simulink model "canLiveReaderModel"  (R2018a)
settings: Solver=FixedStepDiscrete  StartTime=0.0  StopTime=50000  RelTol=1e-3  EnableMultiTasking=on
undefined symbols (not defined in the file or in its folder): canChannel
libraries: simulink x30, canmsglib x15, canlib x5
(part 2 of 2)

== system canLiveReaderModel/CAN Information Output/Targets 0-9/Subsystem/Information Target 8/Check Target Format ==
  CAN Message : Inport
  Compare To Constant1 : simulink/Logic and Bit Operations/Compare To Constant  relop===  const=2  OutDataTypeStr=boolean
  Compare To Constant2 : simulink/Logic and Bit Operations/Compare To Constant  relop===  const=1  OutDataTypeStr=boolean
  Compare To Constant3 : simulink/Logic and Bit Operations/Compare To Constant  relop===  const=3  OutDataTypeStr=boolean
  Divide by 16 : Subsystem
  Selector4 : Selector  IndexMode=Zero-based  InputPortWidth=8  IndexOptions=Index vector (dialog)  Indices=6  OutputSizes=1
  Is format 1? : Outport
  Is format 2? : Outport  Port=2
  Is format 3? : Outport  Port=3
  wires:
  Divide by 16/1(Result) -> Compare To Constant3/1, Compare To Constant2/1, Compare To Constant1/1
  CAN Message/1 -> Selector4/1
  Selector4/1 -> Divide by 16/1(Dividend)
  Compare To Constant1/1 -> Is format 2?/1
  Compare To Constant2/1 -> Is format 1?/1
  Compare To Constant3/1 -> Is format 3?/1

== system canLiveReaderModel/CAN Information Output/Targets 0-9/Subsystem/Information Target 8/Target Format 2 ==
  CAN Message : Inport
  Enable : EnablePort
  Bearing : Subsystem
  Range : Subsystem
  Range (m) : Outport
  Bearing (°) : Outport  Port=2
  wires:
  CAN Message/1 -> Bearing/1(CAN Message), Range/1(CAN Message)
  Range/1(Range (m)) -> Range (m)/1
  Bearing/1(Bearing (°)) -> Bearing (°)/1

== system canLiveReaderModel/CAN Information Output/Targets 0-9/Subsystem/Information Target 9/Check Target Format ==
  CAN Message : Inport
  Compare To Constant1 : simulink/Logic and Bit Operations/Compare To Constant  relop===  const=2  OutDataTypeStr=boolean
  Compare To Constant2 : simulink/Logic and Bit Operations/Compare To Constant  relop===  const=1  OutDataTypeStr=boolean
  Compare To Constant3 : simulink/Logic and Bit Operations/Compare To Constant  relop===  const=3  OutDataTypeStr=boolean
  Divide by 16 : Subsystem
  Selector4 : Selector  IndexMode=Zero-based  InputPortWidth=8  IndexOptions=Index vector (dialog)  Indices=6  OutputSizes=1
  Is format 1? : Outport
  Is format 2? : Outport  Port=2
  Is format 3? : Outport  Port=3
  wires:
  Divide by 16/1(Result) -> Compare To Constant3/1, Compare To Constant2/1, Compare To Constant1/1
  CAN Message/1 -> Selector4/1
  Selector4/1 -> Divide by 16/1(Dividend)
  Compare To Constant1/1 -> Is format 2?/1
  Compare To Constant2/1 -> Is format 1?/1
  Compare To Constant3/1 -> Is format 3?/1

== system canLiveReaderModel/CAN Information Output/Targets 0-9/Subsystem/Information Target 9/Target Format 2 ==
  CAN Message : Inport
  Enable : EnablePort
  Bearing : Subsystem
  Range : Subsystem
  Range (m) : Outport
  Bearing (°) : Outport  Port=2
  wires:
  CAN Message/1 -> Bearing/1(CAN Message), Range/1(CAN Message)
  Range/1(Range (m)) -> Range (m)/1
  Bearing/1(Bearing (°)) -> Bearing (°)/1

== system canLiveReaderModel/CAN Information Output/Targets 0-9/Subsystem/Information Target 0/Check Target Format/Divide by 16 ==
  Dividend : Inport
  Constant1 : Constant  Value=16  OutDataTypeStr=Inherit: Inherit via back propagation
  Divide : Product  Inputs=*/
  Result : Outport
  wires:
  Constant1/1 -> Divide/2
  Dividend/1 -> Divide/1
  Divide/1 -> Result/1

== system canLiveReaderModel/CAN Information Output/Targets 0-9/Subsystem/Information Target 0/Target Format 2/Bearing ==
  CAN Message : Inport
  Divide by 5 : Subsystem
  Gain1 : Gain  Gain=256  OutDataTypeStr=uint16
  Gain2 : Gain  OutDataTypeStr=uint16
  Mod 4 : Subsystem
  Selector2 : Selector  IndexMode=Zero-based  InputPortWidth=8  IndexOptions=Index vector (dialog)  Indices=2  OutputSizes=1
  Selector3 : Selector  IndexMode=Zero-based  InputPortWidth=8  IndexOptions=Index vector (dialog)  Indices=3  OutputSizes=1
  Sum1 : Sum  Inputs=|++|  OutMin=-512  OutMax=511  OutDataTypeStr=fixdt(1,10,0)  InputSameDT=on
  Bearing (°) : Outport
  wires:
  Sum1/1 -> Divide by 5/1(Dividend)
  Gain2/1 -> Sum1/2
  Mod 4/1(Output) -> Gain1/1
  Gain1/1 -> Sum1/1
  CAN Message/1 -> Selector3/1, Selector2/1
  Divide by 5/1(Result) -> Bearing (°)/1
  Selector3/1 -> Gain2/1
  Selector2/1 -> Mod 4/1(Input)

== system canLiveReaderModel/CAN Information Output/Targets 0-9/Subsystem/Information Target 0/Target Format 2/Range ==
  CAN Message : Inport
  Divide by 100 : Subsystem
  Divide by 16 : Subsystem
  Gain : Gain  Gain=16  OutDataTypeStr=uint16
  Selector : Selector  IndexMode=Zero-based  InputPortWidth=8  IndexOptions=Index vector (dialog)  Indices=1  OutputSizes=1
  Selector1 : Selector  IndexMode=Zero-based  InputPortWidth=8  IndexOptions=Index vector (dialog)  Indices=0  OutputSizes=1
  Sum : Sum  Inputs=|++|  AccumDataTypeStr=uint16  InputSameDT=on
  Range (m) : Outport
  wires:
  Selector/1 -> Divide by 16/1(Dividend)
  Sum/1 -> Divide by 100/1(Dividend)
  Divide by 16/1(Result) -> Sum/2
  Divide by 100/1(Result) -> Range (m)/1
  CAN Message/1 -> Selector/1, Selector1/1
  Selector1/1 -> Gain/1
  Gain/1 -> Sum/1

== system canLiveReaderModel/CAN Information Output/Targets 0-9/Subsystem/Information Target 1/Check Target Format/Divide by 16 ==
  Dividend : Inport
  Constant1 : Constant  Value=16  OutDataTypeStr=Inherit: Inherit via back propagation
  Divide : Product  Inputs=*/
  Result : Outport
  wires:
  Constant1/1 -> Divide/2
  Dividend/1 -> Divide/1
  Divide/1 -> Result/1

== system canLiveReaderModel/CAN Information Output/Targets 0-9/Subsystem/Information Target 1/Target Format 2/Bearing ==
  CAN Message : Inport
  Divide by 5 : Subsystem
  Gain1 : Gain  Gain=256  OutDataTypeStr=uint16
  Gain2 : Gain  OutDataTypeStr=uint16
  Mod 4 : Subsystem
  Selector2 : Selector  IndexMode=Zero-based  InputPortWidth=8  IndexOptions=Index vector (dialog)  Indices=2  OutputSizes=1
  Selector3 : Selector  IndexMode=Zero-based  InputPortWidth=8  IndexOptions=Index vector (dialog)  Indices=3  OutputSizes=1
  Sum1 : Sum  Inputs=|++|  OutMin=-512  OutMax=511  OutDataTypeStr=fixdt(1,10,0)  InputSameDT=on
  Bearing (°) : Outport
  wires:
  Sum1/1 -> Divide by 5/1(Dividend)
  Gain2/1 -> Sum1/2
  Mod 4/1(Output) -> Gain1/1
  Gain1/1 -> Sum1/1
  CAN Message/1 -> Selector3/1, Selector2/1
  Divide by 5/1(Result) -> Bearing (°)/1
  Selector3/1 -> Gain2/1
  Selector2/1 -> Mod 4/1(Input)

== system canLiveReaderModel/CAN Information Output/Targets 0-9/Subsystem/Information Target 1/Target Format 2/Range ==
  CAN Message : Inport
  Divide by 100 : Subsystem
  Divide by 16 : Subsystem
  Gain : Gain  Gain=16  OutDataTypeStr=uint16
  Selector : Selector  IndexMode=Zero-based  InputPortWidth=8  IndexOptions=Index vector (dialog)  Indices=1  OutputSizes=1
  Selector1 : Selector  IndexMode=Zero-based  InputPortWidth=8  IndexOptions=Index vector (dialog)  Indices=0  OutputSizes=1
  Sum : Sum  Inputs=|++|  AccumDataTypeStr=uint16  InputSameDT=on
  Range (m) : Outport
  wires:
  Selector/1 -> Divide by 16/1(Dividend)
  Sum/1 -> Divide by 100/1(Dividend)
  Divide by 16/1(Result) -> Sum/2
  Divide by 100/1(Result) -> Range (m)/1
  CAN Message/1 -> Selector/1, Selector1/1
  Selector1/1 -> Gain/1
  Gain/1 -> Sum/1

== system canLiveReaderModel/CAN Information Output/Targets 0-9/Subsystem/Information Target 2/Check Target Format/Divide by 16 ==
  Dividend : Inport
  Constant1 : Constant  Value=16  OutDataTypeStr=Inherit: Inherit via back propagation
  Divide : Product  Inputs=*/
  Result : Outport
  wires:
  Constant1/1 -> Divide/2
  Dividend/1 -> Divide/1
  Divide/1 -> Result/1

== system canLiveReaderModel/CAN Information Output/Targets 0-9/Subsystem/Information Target 2/Target Format 2/Bearing ==
  CAN Message : Inport
  Divide by 5 : Subsystem
  Gain1 : Gain  Gain=256  OutDataTypeStr=uint16
  Gain2 : Gain  OutDataTypeStr=uint16
  Mod 4 : Subsystem
  Selector2 : Selector  IndexMode=Zero-based  InputPortWidth=8  IndexOptions=Index vector (dialog)  Indices=2  OutputSizes=1
  Selector3 : Selector  IndexMode=Zero-based  InputPortWidth=8  IndexOptions=Index vector (dialog)  Indices=3  OutputSizes=1
  Sum1 : Sum  Inputs=|++|  OutMin=-512  OutMax=511  OutDataTypeStr=fixdt(1,10,0)  InputSameDT=on
  Bearing (°) : Outport
  wires:
  Sum1/1 -> Divide by 5/1(Dividend)
  Gain2/1 -> Sum1/2
  Mod 4/1(Output) -> Gain1/1
  Gain1/1 -> Sum1/1
  CAN Message/1 -> Selector3/1, Selector2/1
  Divide by 5/1(Result) -> Bearing (°)/1
  Selector3/1 -> Gain2/1
  Selector2/1 -> Mod 4/1(Input)

== system canLiveReaderModel/CAN Information Output/Targets 0-9/Subsystem/Information Target 2/Target Format 2/Range ==
  CAN Message : Inport
  Divide by 100 : Subsystem
  Divide by 16 : Subsystem
  Gain : Gain  Gain=16  OutDataTypeStr=uint16
  Selector : Selector  IndexMode=Zero-based  InputPortWidth=8  IndexOptions=Index vector (dialog)  Indices=1  OutputSizes=1
  Selector1 : Selector  IndexMode=Zero-based  InputPortWidth=8  IndexOptions=Index vector (dialog)  Indices=0  OutputSizes=1
  Sum : Sum  Inputs=|++|  AccumDataTypeStr=uint16  InputSameDT=on
  Range (m) : Outport
  wires:
  Selector/1 -> Divide by 16/1(Dividend)
  Sum/1 -> Divide by 100/1(Dividend)
  Divide by 16/1(Result) -> Sum/2
  Divide by 100/1(Result) -> Range (m)/1
  CAN Message/1 -> Selector/1, Selector1/1
  Selector1/1 -> Gain/1
  Gain/1 -> Sum/1

== system canLiveReaderModel/CAN Information Output/Targets 0-9/Subsystem/Information Target 3/Check Target Format/Divide by 16 ==
  Dividend : Inport
  Constant1 : Constant  Value=16  OutDataTypeStr=Inherit: Inherit via back propagation
  Divide : Product  Inputs=*/
  Result : Outport
  wires:
  Constant1/1 -> Divide/2
  Dividend/1 -> Divide/1
  Divide/1 -> Result/1

== system canLiveReaderModel/CAN Information Output/Targets 0-9/Subsystem/Information Target 3/Target Format 2/Bearing ==
  CAN Message : Inport
  Divide by 5 : Subsystem
  Gain1 : Gain  Gain=256  OutDataTypeStr=uint16
  Gain2 : Gain  OutDataTypeStr=uint16
  Mod 4 : Subsystem
  Selector2 : Selector  IndexMode=Zero-based  InputPortWidth=8  IndexOptions=Index vector (dialog)  Indices=2  OutputSizes=1
  Selector3 : Selector  IndexMode=Zero-based  InputPortWidth=8  IndexOptions=Index vector (dialog)  Indices=3  OutputSizes=1
  Sum1 : Sum  Inputs=|++|  OutMin=-512  OutMax=511  OutDataTypeStr=fixdt(1,10,0)  InputSameDT=on
  Bearing (°) : Outport
  wires:
  Sum1/1 -> Divide by 5/1(Dividend)
  Gain2/1 -> Sum1/2
  Mod 4/1(Output) -> Gain1/1
  Gain1/1 -> Sum1/1
  CAN Message/1 -> Selector3/1, Selector2/1
  Divide by 5/1(Result) -> Bearing (°)/1
  Selector3/1 -> Gain2/1
  Selector2/1 -> Mod 4/1(Input)

== system canLiveReaderModel/CAN Information Output/Targets 0-9/Subsystem/Information Target 3/Target Format 2/Range ==
  CAN Message : Inport
  Divide by 100 : Subsystem
  Divide by 16 : Subsystem
  Gain : Gain  Gain=16  OutDataTypeStr=uint16
  Selector : Selector  IndexMode=Zero-based  InputPortWidth=8  IndexOptions=Index vector (dialog)  Indices=1  OutputSizes=1
  Selector1 : Selector  IndexMode=Zero-based  InputPortWidth=8  IndexOptions=Index vector (dialog)  Indices=0  OutputSizes=1
  Sum : Sum  Inputs=|++|  AccumDataTypeStr=uint16  InputSameDT=on
  Range (m) : Outport
  wires:
  Selector/1 -> Divide by 16/1(Dividend)
  Sum/1 -> Divide by 100/1(Dividend)
  Divide by 16/1(Result) -> Sum/2
  Divide by 100/1(Result) -> Range (m)/1
  CAN Message/1 -> Selector/1, Selector1/1
  Selector1/1 -> Gain/1
  Gain/1 -> Sum/1

== system canLiveReaderModel/CAN Information Output/Targets 0-9/Subsystem/Information Target 4/Check Target Format/Divide by 16 ==
  Dividend : Inport
  Constant1 : Constant  Value=16  OutDataTypeStr=Inherit: Inherit via back propagation
  Divide : Product  Inputs=*/
  Result : Outport
  wires:
  Constant1/1 -> Divide/2
  Dividend/1 -> Divide/1
  Divide/1 -> Result/1

== system canLiveReaderModel/CAN Information Output/Targets 0-9/Subsystem/Information Target 4/Target Format 2/Bearing ==
  CAN Message : Inport
  Divide by 5 : Subsystem
  Gain1 : Gain  Gain=256  OutDataTypeStr=uint16
  Gain2 : Gain  OutDataTypeStr=uint16
  Mod 4 : Subsystem
  Selector2 : Selector  IndexMode=Zero-based  InputPortWidth=8  IndexOptions=Index vector (dialog)  Indices=2  OutputSizes=1
  Selector3 : Selector  IndexMode=Zero-based  InputPortWidth=8  IndexOptions=Index vector (dialog)  Indices=3  OutputSizes=1
  Sum1 : Sum  Inputs=|++|  OutMin=-512  OutMax=511  OutDataTypeStr=fixdt(1,10,0)  InputSameDT=on
  Bearing (°) : Outport
  wires:
  Sum1/1 -> Divide by 5/1(Dividend)
  Gain2/1 -> Sum1/2
  Mod 4/1(Output) -> Gain1/1
  Gain1/1 -> Sum1/1
  CAN Message/1 -> Selector3/1, Selector2/1
  Divide by 5/1(Result) -> Bearing (°)/1
  Selector3/1 -> Gain2/1
  Selector2/1 -> Mod 4/1(Input)

== system canLiveReaderModel/CAN Information Output/Targets 0-9/Subsystem/Information Target 4/Target Format 2/Range ==
  CAN Message : Inport
  Divide by 100 : Subsystem
  Divide by 16 : Subsystem
  Gain : Gain  Gain=16  OutDataTypeStr=uint16
  Selector : Selector  IndexMode=Zero-based  InputPortWidth=8  IndexOptions=Index vector (dialog)  Indices=1  OutputSizes=1
  Selector1 : Selector  IndexMode=Zero-based  InputPortWidth=8  IndexOptions=Index vector (dialog)  Indices=0  OutputSizes=1
  Sum : Sum  Inputs=|++|  AccumDataTypeStr=uint16  InputSameDT=on
  Range (m) : Outport
  wires:
  Selector/1 -> Divide by 16/1(Dividend)
  Sum/1 -> Divide by 100/1(Dividend)
  Divide by 16/1(Result) -> Sum/2
  Divide by 100/1(Result) -> Range (m)/1
  CAN Message/1 -> Selector/1, Selector1/1
  Selector1/1 -> Gain/1
  Gain/1 -> Sum/1

== system canLiveReaderModel/CAN Information Output/Targets 0-9/Subsystem/Information Target 5/Check Target Format/Divide by 16 ==
  Dividend : Inport
  Constant1 : Constant  Value=16  OutDataTypeStr=Inherit: Inherit via back propagation
  Divide : Product  Inputs=*/
  Result : Outport
  wires:
  Constant1/1 -> Divide/2
  Dividend/1 -> Divide/1
  Divide/1 -> Result/1

== system canLiveReaderModel/CAN Information Output/Targets 0-9/Subsystem/Information Target 5/Target Format 2/Bearing ==
  CAN Message : Inport
  Divide by 5 : Subsystem
  Gain1 : Gain  Gain=256  OutDataTypeStr=uint16
  Gain2 : Gain  OutDataTypeStr=uint16
  Mod 4 : Subsystem
  Selector2 : Selector  IndexMode=Zero-based  InputPortWidth=8  IndexOptions=Index vector (dialog)  Indices=2  OutputSizes=1
  Selector3 : Selector  IndexMode=Zero-based  InputPortWidth=8  IndexOptions=Index vector (dialog)  Indices=3  OutputSizes=1
  Sum1 : Sum  Inputs=|++|  OutMin=-512  OutMax=511  OutDataTypeStr=fixdt(1,10,0)  InputSameDT=on
  Bearing (°) : Outport
  wires:
  Sum1/1 -> Divide by 5/1(Dividend)
  Gain2/1 -> Sum1/2
  Mod 4/1(Output) -> Gain1/1
  Gain1/1 -> Sum1/1
  CAN Message/1 -> Selector3/1, Selector2/1
  Divide by 5/1(Result) -> Bearing (°)/1
  Selector3/1 -> Gain2/1
  Selector2/1 -> Mod 4/1(Input)

== system canLiveReaderModel/CAN Information Output/Targets 0-9/Subsystem/Information Target 5/Target Format 2/Range ==
  CAN Message : Inport
  Divide by 100 : Subsystem
  Divide by 16 : Subsystem
  Gain : Gain  Gain=16  OutDataTypeStr=uint16
  Selector : Selector  IndexMode=Zero-based  InputPortWidth=8  IndexOptions=Index vector (dialog)  Indices=1  OutputSizes=1
  Selector1 : Selector  IndexMode=Zero-based  InputPortWidth=8  IndexOptions=Index vector (dialog)  Indices=0  OutputSizes=1
  Sum : Sum  Inputs=|++|  AccumDataTypeStr=uint16  InputSameDT=on
  Range (m) : Outport
  wires:
  Selector/1 -> Divide by 16/1(Dividend)
  Sum/1 -> Divide by 100/1(Dividend)
  Divide by 16/1(Result) -> Sum/2
  Divide by 100/1(Result) -> Range (m)/1
  CAN Message/1 -> Selector/1, Selector1/1
  Selector1/1 -> Gain/1
  Gain/1 -> Sum/1

== system canLiveReaderModel/CAN Information Output/Targets 0-9/Subsystem/Information Target 6/Check Target Format/Divide by 16 ==
  Dividend : Inport
  Constant1 : Constant  Value=16  OutDataTypeStr=Inherit: Inherit via back propagation
  Divide : Product  Inputs=*/
  Result : Outport
  wires:
  Constant1/1 -> Divide/2
  Dividend/1 -> Divide/1
  Divide/1 -> Result/1

== system canLiveReaderModel/CAN Information Output/Targets 0-9/Subsystem/Information Target 6/Target Format 2/Bearing ==
  CAN Message : Inport
  Divide by 5 : Subsystem
  Gain1 : Gain  Gain=256  OutDataTypeStr=uint16
  Gain2 : Gain  OutDataTypeStr=uint16
  Mod 4 : Subsystem
  Selector2 : Selector  IndexMode=Zero-based  InputPortWidth=8  IndexOptions=Index vector (dialog)  Indices=2  OutputSizes=1
  Selector3 : Selector  IndexMode=Zero-based  InputPortWidth=8  IndexOptions=Index vector (dialog)  Indices=3  OutputSizes=1
  Sum1 : Sum  Inputs=|++|  OutMin=-512  OutMax=511  OutDataTypeStr=fixdt(1,10,0)  InputSameDT=on
  Bearing (°) : Outport
  wires:
  Sum1/1 -> Divide by 5/1(Dividend)
  Gain2/1 -> Sum1/2
  Mod 4/1(Output) -> Gain1/1
  Gain1/1 -> Sum1/1
  CAN Message/1 -> Selector3/1, Selector2/1
  Divide by 5/1(Result) -> Bearing (°)/1
  Selector3/1 -> Gain2/1
  Selector2/1 -> Mod 4/1(Input)

== system canLiveReaderModel/CAN Information Output/Targets 0-9/Subsystem/Information Target 6/Target Format 2/Range ==
  CAN Message : Inport
  Divide by 100 : Subsystem
  Divide by 16 : Subsystem
  Gain : Gain  Gain=16  OutDataTypeStr=uint16
  Selector : Selector  IndexMode=Zero-based  InputPortWidth=8  IndexOptions=Index vector (dialog)  Indices=1  OutputSizes=1
  Selector1 : Selector  IndexMode=Zero-based  InputPortWidth=8  IndexOptions=Index vector (dialog)  Indices=0  OutputSizes=1
  Sum : Sum  Inputs=|++|  AccumDataTypeStr=uint16  InputSameDT=on
  Range (m) : Outport
  wires:
  Selector/1 -> Divide by 16/1(Dividend)
  Sum/1 -> Divide by 100/1(Dividend)
  Divide by 16/1(Result) -> Sum/2
  Divide by 100/1(Result) -> Range (m)/1
  CAN Message/1 -> Selector/1, Selector1/1
  Selector1/1 -> Gain/1
  Gain/1 -> Sum/1

== system canLiveReaderModel/CAN Information Output/Targets 0-9/Subsystem/Information Target 7/Check Target Format/Divide by 16 ==
  Dividend : Inport
  Constant1 : Constant  Value=16  OutDataTypeStr=Inherit: Inherit via back propagation
  Divide : Product  Inputs=*/
  Result : Outport
  wires:
  Constant1/1 -> Divide/2
  Dividend/1 -> Divide/1
  Divide/1 -> Result/1

== system canLiveReaderModel/CAN Information Output/Targets 0-9/Subsystem/Information Target 7/Target Format 2/Bearing ==
  CAN Message : Inport
  Divide by 5 : Subsystem
  Gain1 : Gain  Gain=256  OutDataTypeStr=uint16
  Gain2 : Gain  OutDataTypeStr=uint16
  Mod 4 : Subsystem
  Selector2 : Selector  IndexMode=Zero-based  InputPortWidth=8  IndexOptions=Index vector (dialog)  Indices=2  OutputSizes=1
  Selector3 : Selector  IndexMode=Zero-based  InputPortWidth=8  IndexOptions=Index vector (dialog)  Indices=3  OutputSizes=1
  Sum1 : Sum  Inputs=|++|  OutMin=-512  OutMax=511  OutDataTypeStr=fixdt(1,10,0)  InputSameDT=on
  Bearing (°) : Outport
  wires:
  Sum1/1 -> Divide by 5/1(Dividend)
  Gain2/1 -> Sum1/2
  Mod 4/1(Output) -> Gain1/1
  Gain1/1 -> Sum1/1
  CAN Message/1 -> Selector3/1, Selector2/1
  Divide by 5/1(Result) -> Bearing (°)/1
  Selector3/1 -> Gain2/1
  Selector2/1 -> Mod 4/1(Input)

== system canLiveReaderModel/CAN Information Output/Targets 0-9/Subsystem/Information Target 7/Target Format 2/Range ==
  CAN Message : Inport
  Divide by 100 : Subsystem
  Divide by 16 : Subsystem
  Gain : Gain  Gain=16  OutDataTypeStr=uint16
  Selector : Selector  IndexMode=Zero-based  InputPortWidth=8  IndexOptions=Index vector (dialog)  Indices=1  OutputSizes=1
  Selector1 : Selector  IndexMode=Zero-based  InputPortWidth=8  IndexOptions=Index vector (dialog)  Indices=0  OutputSizes=1
  Sum : Sum  Inputs=|++|  AccumDataTypeStr=uint16  InputSameDT=on
  Range (m) : Outport
  wires:
  Selector/1 -> Divide by 16/1(Dividend)
  Sum/1 -> Divide by 100/1(Dividend)
  Divide by 16/1(Result) -> Sum/2
  Divide by 100/1(Result) -> Range (m)/1
  CAN Message/1 -> Selector/1, Selector1/1
  Selector1/1 -> Gain/1
  Gain/1 -> Sum/1

== system canLiveReaderModel/CAN Information Output/Targets 0-9/Subsystem/Information Target 8/Check Target Format/Divide by 16 ==
  Dividend : Inport
  Constant1 : Constant  Value=16  OutDataTypeStr=Inherit: Inherit via back propagation
  Divide : Product  Inputs=*/
  Result : Outport
  wires:
  Constant1/1 -> Divide/2
  Dividend/1 -> Divide/1
  Divide/1 -> Result/1

== system canLiveReaderModel/CAN Information Output/Targets 0-9/Subsystem/Information Target 8/Target Format 2/Bearing ==
  CAN Message : Inport
  Divide by 5 : Subsystem
  Gain1 : Gain  Gain=256  OutDataTypeStr=uint16
  Gain2 : Gain  OutDataTypeStr=uint16
  Mod 4 : Subsystem
  Selector2 : Selector  IndexMode=Zero-based  InputPortWidth=8  IndexOptions=Index vector (dialog)  Indices=2  OutputSizes=1
  Selector3 : Selector  IndexMode=Zero-based  InputPortWidth=8  IndexOptions=Index vector (dialog)  Indices=3  OutputSizes=1
  Sum1 : Sum  Inputs=|++|  OutMin=-512  OutMax=511  OutDataTypeStr=fixdt(1,10,0)  InputSameDT=on
  Bearing (°) : Outport
  wires:
  Sum1/1 -> Divide by 5/1(Dividend)
  Gain2/1 -> Sum1/2
  Mod 4/1(Output) -> Gain1/1
  Gain1/1 -> Sum1/1
  CAN Message/1 -> Selector3/1, Selector2/1
  Divide by 5/1(Result) -> Bearing (°)/1
  Selector3/1 -> Gain2/1
  Selector2/1 -> Mod 4/1(Input)

== system canLiveReaderModel/CAN Information Output/Targets 0-9/Subsystem/Information Target 8/Target Format 2/Range ==
  CAN Message : Inport
  Divide by 100 : Subsystem
  Divide by 16 : Subsystem
  Gain : Gain  Gain=16  OutDataTypeStr=uint16
  Selector : Selector  IndexMode=Zero-based  InputPortWidth=8  IndexOptions=Index vector (dialog)  Indices=1  OutputSizes=1
  Selector1 : Selector  IndexMode=Zero-based  InputPortWidth=8  IndexOptions=Index vector (dialog)  Indices=0  OutputSizes=1
  Sum : Sum  Inputs=|++|  AccumDataTypeStr=uint16  InputSameDT=on
  Range (m) : Outport
  wires:
  Selector/1 -> Divide by 16/1(Dividend)
  Sum/1 -> Divide by 100/1(Dividend)
  Divide by 16/1(Result) -> Sum/2
  Divide by 100/1(Result) -> Range (m)/1
  CAN Message/1 -> Selector/1, Selector1/1
  Selector1/1 -> Gain/1
  Gain/1 -> Sum/1

== system canLiveReaderModel/CAN Information Output/Targets 0-9/Subsystem/Information Target 9/Check Target Format/Divide by 16 ==
  Dividend : Inport
  Constant1 : Constant  Value=16  OutDataTypeStr=Inherit: Inherit via back propagation
  Divide : Product  Inputs=*/
  Result : Outport
  wires:
  Constant1/1 -> Divide/2
  Dividend/1 -> Divide/1
  Divide/1 -> Result/1

== system canLiveReaderModel/CAN Information Output/Targets 0-9/Subsystem/Information Target 9/Target Format 2/Bearing ==
  CAN Message : Inport
  Divide by 5 : Subsystem
  Gain1 : Gain  Gain=256  OutDataTypeStr=uint16
  Gain2 : Gain  OutDataTypeStr=uint16
  Mod 4 : Subsystem
  Selector2 : Selector  IndexMode=Zero-based  InputPortWidth=8  IndexOptions=Index vector (dialog)  Indices=2  OutputSizes=1
  Selector3 : Selector  IndexMode=Zero-based  InputPortWidth=8  IndexOptions=Index vector (dialog)  Indices=3  OutputSizes=1
  Sum1 : Sum  Inputs=|++|  OutMin=-512  OutMax=511  OutDataTypeStr=fixdt(1,10,0)  InputSameDT=on
  Bearing (°) : Outport
  wires:
  Sum1/1 -> Divide by 5/1(Dividend)
  Gain2/1 -> Sum1/2
  Mod 4/1(Output) -> Gain1/1
  Gain1/1 -> Sum1/1
  CAN Message/1 -> Selector3/1, Selector2/1
  Divide by 5/1(Result) -> Bearing (°)/1
  Selector3/1 -> Gain2/1
  Selector2/1 -> Mod 4/1(Input)

== system canLiveReaderModel/CAN Information Output/Targets 0-9/Subsystem/Information Target 9/Target Format 2/Range ==
  CAN Message : Inport
  Divide by 100 : Subsystem
  Divide by 16 : Subsystem
  Gain : Gain  Gain=16  OutDataTypeStr=uint16
  Selector : Selector  IndexMode=Zero-based  InputPortWidth=8  IndexOptions=Index vector (dialog)  Indices=1  OutputSizes=1
  Selector1 : Selector  IndexMode=Zero-based  InputPortWidth=8  IndexOptions=Index vector (dialog)  Indices=0  OutputSizes=1
  Sum : Sum  Inputs=|++|  AccumDataTypeStr=uint16  InputSameDT=on
  Range (m) : Outport
  wires:
  Selector/1 -> Divide by 16/1(Dividend)
  Sum/1 -> Divide by 100/1(Dividend)
  Divide by 16/1(Result) -> Sum/2
  Divide by 100/1(Result) -> Range (m)/1
  CAN Message/1 -> Selector/1, Selector1/1
  Selector1/1 -> Gain/1
  Gain/1 -> Sum/1

== system canLiveReaderModel/CAN Information Output/Targets 0-9/Subsystem/Information Target 0/Target Format 2/Bearing/Divide by 5 ==
  Dividend : Inport
  Constant1 : Constant  Value=5  OutDataTypeStr=Inherit: Inherit via back propagation
  Divide : Product  Inputs=*/  OutDataTypeStr=double
  Result : Outport
  wires:
  Constant1/1 -> Divide/2
  Divide/1 -> Result/1
  Dividend/1 -> Divide/1

== system canLiveReaderModel/CAN Information Output/Targets 0-9/Subsystem/Information Target 0/Target Format 2/Bearing/Mod 4 ==
  Input : Inport
  Constant : Constant  Value=4  OutDataTypeStr=Inherit: Inherit via back propagation
  Rem : Math  Operator=mod  OutputSignalType=real  SaturateOnIntegerOverflow=on
  Output : Outport
  wires:
  Input/1 -> Rem/1
  Constant/1 -> Rem/2
  Rem/1 -> Output/1

== system canLiveReaderModel/CAN Information Output/Targets 0-9/Subsystem/Information Target 0/Target Format 2/Range/Divide by 100 ==
  Dividend : Inport
  Constant1 : Constant  Value=100  OutDataTypeStr=Inherit: Inherit via back propagation
  Divide : Product  Inputs=*/  OutDataTypeStr=double
  Result : Outport
  wires:
  Constant1/1 -> Divide/2
  Divide/1 -> Result/1
  Dividend/1 -> Divide/1

== system canLiveReaderModel/CAN Information Output/Targets 0-9/Subsystem/Information Target 0/Target Format 2/Range/Divide by 16 ==
  Dividend : Inport
  Constant1 : Constant  Value=16  OutDataTypeStr=Inherit: Inherit via back propagation
  Divide : Product  Inputs=*/
  Result : Outport
  wires:
  Constant1/1 -> Divide/2
  Dividend/1 -> Divide/1
  Divide/1 -> Result/1

== system canLiveReaderModel/CAN Information Output/Targets 0-9/Subsystem/Information Target 1/Target Format 2/Bearing/Divide by 5 ==
  Dividend : Inport
  Constant1 : Constant  Value=5  OutDataTypeStr=Inherit: Inherit via back propagation
  Divide : Product  Inputs=*/  OutDataTypeStr=double
  Result : Outport
  wires:
  Constant1/1 -> Divide/2
  Divide/1 -> Result/1
  Dividend/1 -> Divide/1

== system canLiveReaderModel/CAN Information Output/Targets 0-9/Subsystem/Information Target 1/Target Format 2/Bearing/Mod 4 ==
  Input : Inport
  Constant : Constant  Value=4  OutDataTypeStr=Inherit: Inherit via back propagation
  Rem : Math  Operator=mod  OutputSignalType=real  SaturateOnIntegerOverflow=on
  Output : Outport
  wires:
  Input/1 -> Rem/1
  Constant/1 -> Rem/2
  Rem/1 -> Output/1

== system canLiveReaderModel/CAN Information Output/Targets 0-9/Subsystem/Information Target 1/Target Format 2/Range/Divide by 100 ==
  Dividend : Inport
  Constant1 : Constant  Value=100  OutDataTypeStr=Inherit: Inherit via back propagation
  Divide : Product  Inputs=*/  OutDataTypeStr=double
  Result : Outport
  wires:
  Constant1/1 -> Divide/2
  Divide/1 -> Result/1
  Dividend/1 -> Divide/1

== system canLiveReaderModel/CAN Information Output/Targets 0-9/Subsystem/Information Target 1/Target Format 2/Range/Divide by 16 ==
  Dividend : Inport
  Constant1 : Constant  Value=16  OutDataTypeStr=Inherit: Inherit via back propagation
  Divide : Product  Inputs=*/
  Result : Outport
  wires:
  Constant1/1 -> Divide/2
  Dividend/1 -> Divide/1
  Divide/1 -> Result/1

== system canLiveReaderModel/CAN Information Output/Targets 0-9/Subsystem/Information Target 2/Target Format 2/Bearing/Divide by 5 ==
  Dividend : Inport
  Constant1 : Constant  Value=5  OutDataTypeStr=Inherit: Inherit via back propagation
  Divide : Product  Inputs=*/  OutDataTypeStr=double
  Result : Outport
  wires:
  Constant1/1 -> Divide/2
  Divide/1 -> Result/1
  Dividend/1 -> Divide/1

== system canLiveReaderModel/CAN Information Output/Targets 0-9/Subsystem/Information Target 2/Target Format 2/Bearing/Mod 4 ==
  Input : Inport
  Constant : Constant  Value=4  OutDataTypeStr=Inherit: Inherit via back propagation
  Rem : Math  Operator=mod  OutputSignalType=real  SaturateOnIntegerOverflow=on
  Output : Outport
  wires:
  Input/1 -> Rem/1
  Constant/1 -> Rem/2
  Rem/1 -> Output/1

== system canLiveReaderModel/CAN Information Output/Targets 0-9/Subsystem/Information Target 2/Target Format 2/Range/Divide by 100 ==
  Dividend : Inport
  Constant1 : Constant  Value=100  OutDataTypeStr=Inherit: Inherit via back propagation
  Divide : Product  Inputs=*/  OutDataTypeStr=double
  Result : Outport
  wires:
  Constant1/1 -> Divide/2
  Divide/1 -> Result/1
  Dividend/1 -> Divide/1

== system canLiveReaderModel/CAN Information Output/Targets 0-9/Subsystem/Information Target 2/Target Format 2/Range/Divide by 16 ==
  Dividend : Inport
  Constant1 : Constant  Value=16  OutDataTypeStr=Inherit: Inherit via back propagation
  Divide : Product  Inputs=*/
  Result : Outport
  wires:
  Constant1/1 -> Divide/2
  Dividend/1 -> Divide/1
  Divide/1 -> Result/1

== system canLiveReaderModel/CAN Information Output/Targets 0-9/Subsystem/Information Target 3/Target Format 2/Bearing/Divide by 5 ==
  Dividend : Inport
  Constant1 : Constant  Value=5  OutDataTypeStr=Inherit: Inherit via back propagation
  Divide : Product  Inputs=*/  OutDataTypeStr=double
  Result : Outport
  wires:
  Constant1/1 -> Divide/2
  Divide/1 -> Result/1
  Dividend/1 -> Divide/1

== system canLiveReaderModel/CAN Information Output/Targets 0-9/Subsystem/Information Target 3/Target Format 2/Bearing/Mod 4 ==
  Input : Inport
  Constant : Constant  Value=4  OutDataTypeStr=Inherit: Inherit via back propagation
  Rem : Math  Operator=mod  OutputSignalType=real  SaturateOnIntegerOverflow=on
  Output : Outport
  wires:
  Input/1 -> Rem/1
  Constant/1 -> Rem/2
  Rem/1 -> Output/1

== system canLiveReaderModel/CAN Information Output/Targets 0-9/Subsystem/Information Target 3/Target Format 2/Range/Divide by 100 ==
  Dividend : Inport
  Constant1 : Constant  Value=100  OutDataTypeStr=Inherit: Inherit via back propagation
  Divide : Product  Inputs=*/  OutDataTypeStr=double
  Result : Outport
  wires:
  Constant1/1 -> Divide/2
  Divide/1 -> Result/1
  Dividend/1 -> Divide/1

== system canLiveReaderModel/CAN Information Output/Targets 0-9/Subsystem/Information Target 3/Target Format 2/Range/Divide by 16 ==
  Dividend : Inport
  Constant1 : Constant  Value=16  OutDataTypeStr=Inherit: Inherit via back propagation
  Divide : Product  Inputs=*/
  Result : Outport
  wires:
  Constant1/1 -> Divide/2
  Dividend/1 -> Divide/1
  Divide/1 -> Result/1

== system canLiveReaderModel/CAN Information Output/Targets 0-9/Subsystem/Information Target 4/Target Format 2/Bearing/Divide by 5 ==
  Dividend : Inport
  Constant1 : Constant  Value=5  OutDataTypeStr=Inherit: Inherit via back propagation
  Divide : Product  Inputs=*/  OutDataTypeStr=double
  Result : Outport
  wires:
  Constant1/1 -> Divide/2
  Divide/1 -> Result/1
  Dividend/1 -> Divide/1

== system canLiveReaderModel/CAN Information Output/Targets 0-9/Subsystem/Information Target 4/Target Format 2/Bearing/Mod 4 ==
  Input : Inport
  Constant : Constant  Value=4  OutDataTypeStr=Inherit: Inherit via back propagation
  Rem : Math  Operator=mod  OutputSignalType=real  SaturateOnIntegerOverflow=on
  Output : Outport
  wires:
  Input/1 -> Rem/1
  Constant/1 -> Rem/2
  Rem/1 -> Output/1

== system canLiveReaderModel/CAN Information Output/Targets 0-9/Subsystem/Information Target 4/Target Format 2/Range/Divide by 100 ==
  Dividend : Inport
  Constant1 : Constant  Value=100  OutDataTypeStr=Inherit: Inherit via back propagation
  Divide : Product  Inputs=*/  OutDataTypeStr=double
  Result : Outport
  wires:
  Constant1/1 -> Divide/2
  Divide/1 -> Result/1
  Dividend/1 -> Divide/1

== system canLiveReaderModel/CAN Information Output/Targets 0-9/Subsystem/Information Target 4/Target Format 2/Range/Divide by 16 ==
  Dividend : Inport
  Constant1 : Constant  Value=16  OutDataTypeStr=Inherit: Inherit via back propagation
  Divide : Product  Inputs=*/
  Result : Outport
  wires:
  Constant1/1 -> Divide/2
  Dividend/1 -> Divide/1
  Divide/1 -> Result/1

== system canLiveReaderModel/CAN Information Output/Targets 0-9/Subsystem/Information Target 5/Target Format 2/Bearing/Divide by 5 ==
  Dividend : Inport
  Constant1 : Constant  Value=5  OutDataTypeStr=Inherit: Inherit via back propagation
  Divide : Product  Inputs=*/  OutDataTypeStr=double
  Result : Outport
  wires:
  Constant1/1 -> Divide/2
  Divide/1 -> Result/1
  Dividend/1 -> Divide/1

== system canLiveReaderModel/CAN Information Output/Targets 0-9/Subsystem/Information Target 5/Target Format 2/Bearing/Mod 4 ==
  Input : Inport
  Constant : Constant  Value=4  OutDataTypeStr=Inherit: Inherit via back propagation
  Rem : Math  Operator=mod  OutputSignalType=real  SaturateOnIntegerOverflow=on
  Output : Outport
  wires:
  Input/1 -> Rem/1
  Constant/1 -> Rem/2
  Rem/1 -> Output/1

== system canLiveReaderModel/CAN Information Output/Targets 0-9/Subsystem/Information Target 5/Target Format 2/Range/Divide by 100 ==
  Dividend : Inport
  Constant1 : Constant  Value=100  OutDataTypeStr=Inherit: Inherit via back propagation
  Divide : Product  Inputs=*/  OutDataTypeStr=double
  Result : Outport
  wires:
  Constant1/1 -> Divide/2
  Divide/1 -> Result/1
  Dividend/1 -> Divide/1

== system canLiveReaderModel/CAN Information Output/Targets 0-9/Subsystem/Information Target 5/Target Format 2/Range/Divide by 16 ==
  Dividend : Inport
  Constant1 : Constant  Value=16  OutDataTypeStr=Inherit: Inherit via back propagation
  Divide : Product  Inputs=*/
  Result : Outport
  wires:
  Constant1/1 -> Divide/2
  Dividend/1 -> Divide/1
  Divide/1 -> Result/1

== system canLiveReaderModel/CAN Information Output/Targets 0-9/Subsystem/Information Target 6/Target Format 2/Bearing/Divide by 5 ==
  Dividend : Inport
  Constant1 : Constant  Value=5  OutDataTypeStr=Inherit: Inherit via back propagation
  Divide : Product  Inputs=*/  OutDataTypeStr=double
  Result : Outport
  wires:
  Constant1/1 -> Divide/2
  Divide/1 -> Result/1
  Dividend/1 -> Divide/1

== system canLiveReaderModel/CAN Information Output/Targets 0-9/Subsystem/Information Target 6/Target Format 2/Bearing/Mod 4 ==
  Input : Inport
  Constant : Constant  Value=4  OutDataTypeStr=Inherit: Inherit via back propagation
  Rem : Math  Operator=mod  OutputSignalType=real  SaturateOnIntegerOverflow=on
  Output : Outport
  wires:
  Input/1 -> Rem/1
  Constant/1 -> Rem/2
  Rem/1 -> Output/1

== system canLiveReaderModel/CAN Information Output/Targets 0-9/Subsystem/Information Target 6/Target Format 2/Range/Divide by 100 ==
  Dividend : Inport
  Constant1 : Constant  Value=100  OutDataTypeStr=Inherit: Inherit via back propagation
  Divide : Product  Inputs=*/  OutDataTypeStr=double
  Result : Outport
  wires:
  Constant1/1 -> Divide/2
  Divide/1 -> Result/1
  Dividend/1 -> Divide/1

== system canLiveReaderModel/CAN Information Output/Targets 0-9/Subsystem/Information Target 6/Target Format 2/Range/Divide by 16 ==
  Dividend : Inport
  Constant1 : Constant  Value=16  OutDataTypeStr=Inherit: Inherit via back propagation
  Divide : Product  Inputs=*/
  Result : Outport
  wires:
  Constant1/1 -> Divide/2
  Dividend/1 -> Divide/1
  Divide/1 -> Result/1

== system canLiveReaderModel/CAN Information Output/Targets 0-9/Subsystem/Information Target 7/Target Format 2/Bearing/Divide by 5 ==
  Dividend : Inport
  Constant1 : Constant  Value=5  OutDataTypeStr=Inherit: Inherit via back propagation
  Divide : Product  Inputs=*/  OutDataTypeStr=double
  Result : Outport
  wires:
  Constant1/1 -> Divide/2
  Divide/1 -> Result/1
  Dividend/1 -> Divide/1

== system canLiveReaderModel/CAN Information Output/Targets 0-9/Subsystem/Information Target 7/Target Format 2/Bearing/Mod 4 ==
  Input : Inport
  Constant : Constant  Value=4  OutDataTypeStr=Inherit: Inherit via back propagation
  Rem : Math  Operator=mod  OutputSignalType=real  SaturateOnIntegerOverflow=on
  Output : Outport
  wires:
  Input/1 -> Rem/1
  Constant/1 -> Rem/2
  Rem/1 -> Output/1

== system canLiveReaderModel/CAN Information Output/Targets 0-9/Subsystem/Information Target 7/Target Format 2/Range/Divide by 100 ==
  Dividend : Inport
  Constant1 : Constant  Value=100  OutDataTypeStr=Inherit: Inherit via back propagation
  Divide : Product  Inputs=*/  OutDataTypeStr=double
  Result : Outport
  wires:
  Constant1/1 -> Divide/2
  Divide/1 -> Result/1
  Dividend/1 -> Divide/1

== system canLiveReaderModel/CAN Information Output/Targets 0-9/Subsystem/Information Target 7/Target Format 2/Range/Divide by 16 ==
  Dividend : Inport
  Constant1 : Constant  Value=16  OutDataTypeStr=Inherit: Inherit via back propagation
  Divide : Product  Inputs=*/
  Result : Outport
  wires:
  Constant1/1 -> Divide/2
  Dividend/1 -> Divide/1
  Divide/1 -> Result/1

== system canLiveReaderModel/CAN Information Output/Targets 0-9/Subsystem/Information Target 8/Target Format 2/Bearing/Divide by 5 ==
  Dividend : Inport
  Constant1 : Constant  Value=5  OutDataTypeStr=Inherit: Inherit via back propagation
  Divide : Product  Inputs=*/  OutDataTypeStr=double
  Result : Outport
  wires:
  Constant1/1 -> Divide/2
  Divide/1 -> Result/1
  Dividend/1 -> Divide/1

== system canLiveReaderModel/CAN Information Output/Targets 0-9/Subsystem/Information Target 8/Target Format 2/Bearing/Mod 4 ==
  Input : Inport
  Constant : Constant  Value=4  OutDataTypeStr=Inherit: Inherit via back propagation
  Rem : Math  Operator=mod  OutputSignalType=real  SaturateOnIntegerOverflow=on
  Output : Outport
  wires:
  Input/1 -> Rem/1
  Constant/1 -> Rem/2
  Rem/1 -> Output/1

== system canLiveReaderModel/CAN Information Output/Targets 0-9/Subsystem/Information Target 8/Target Format 2/Range/Divide by 100 ==
  Dividend : Inport
  Constant1 : Constant  Value=100  OutDataTypeStr=Inherit: Inherit via back propagation
  Divide : Product  Inputs=*/  OutDataTypeStr=double
  Result : Outport
  wires:
  Constant1/1 -> Divide/2
  Divide/1 -> Result/1
  Dividend/1 -> Divide/1

== system canLiveReaderModel/CAN Information Output/Targets 0-9/Subsystem/Information Target 8/Target Format 2/Range/Divide by 16 ==
  Dividend : Inport
  Constant1 : Constant  Value=16  OutDataTypeStr=Inherit: Inherit via back propagation
  Divide : Product  Inputs=*/
  Result : Outport
  wires:
  Constant1/1 -> Divide/2
  Dividend/1 -> Divide/1
  Divide/1 -> Result/1

== system canLiveReaderModel/CAN Information Output/Targets 0-9/Subsystem/Information Target 9/Target Format 2/Bearing/Divide by 5 ==
  Dividend : Inport
  Constant1 : Constant  Value=5  OutDataTypeStr=Inherit: Inherit via back propagation
  Divide : Product  Inputs=*/  OutDataTypeStr=double
  Result : Outport
  wires:
  Constant1/1 -> Divide/2
  Divide/1 -> Result/1
  Dividend/1 -> Divide/1

== system canLiveReaderModel/CAN Information Output/Targets 0-9/Subsystem/Information Target 9/Target Format 2/Bearing/Mod 4 ==
  Input : Inport
  Constant : Constant  Value=4  OutDataTypeStr=Inherit: Inherit via back propagation
  Rem : Math  Operator=mod  OutputSignalType=real  SaturateOnIntegerOverflow=on
  Output : Outport
  wires:
  Input/1 -> Rem/1
  Constant/1 -> Rem/2
  Rem/1 -> Output/1

== system canLiveReaderModel/CAN Information Output/Targets 0-9/Subsystem/Information Target 9/Target Format 2/Range/Divide by 100 ==
  Dividend : Inport
  Constant1 : Constant  Value=100  OutDataTypeStr=Inherit: Inherit via back propagation
  Divide : Product  Inputs=*/  OutDataTypeStr=double
  Result : Outport
  wires:
  Constant1/1 -> Divide/2
  Divide/1 -> Result/1
  Dividend/1 -> Divide/1

== system canLiveReaderModel/CAN Information Output/Targets 0-9/Subsystem/Information Target 9/Target Format 2/Range/Divide by 16 ==
  Dividend : Inport
  Constant1 : Constant  Value=16  OutDataTypeStr=Inherit: Inherit via back propagation
  Divide : Product  Inputs=*/
  Result : Outport
  wires:
  Constant1/1 -> Divide/2
  Dividend/1 -> Divide/1
  Divide/1 -> Result/1
